simulink model "sampleModel1455"  (R2023a)
settings: Solver=VariableStepAuto  StartTime=0.0  StopTime=10.0  RelTol=1e-3
libraries: hdlsllib x5, simulink x3
settings Model: Creator=user1  LastModifiedBy=user1

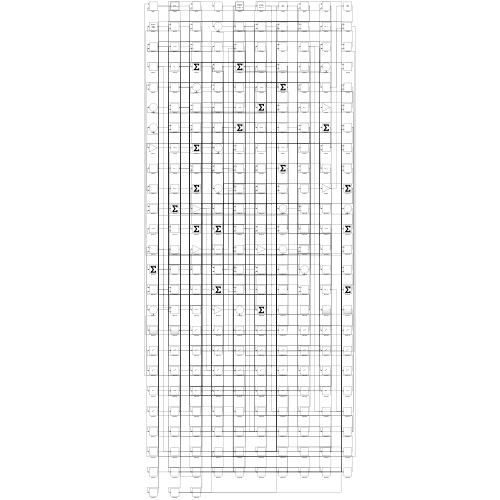
[thumbnail: Simulink's stored preview of the top-level diagram]
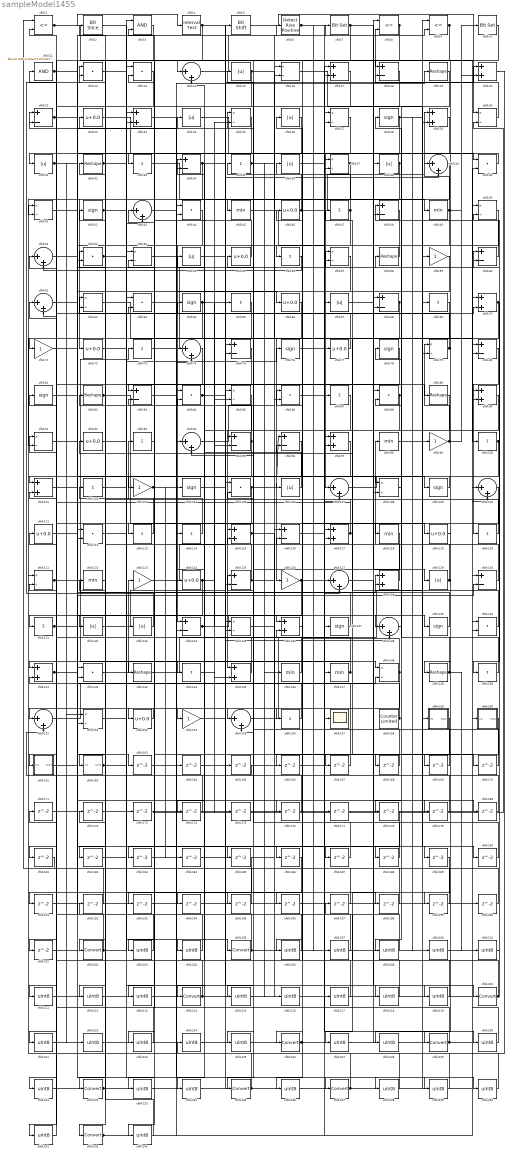
== system sampleModel1455 ==
  cfblk1 : RelationalOperator  Operator=<=  OutDataTypeStr=boolean  InputSameDT=off
  cfblk10 : simulink/Logic and Bit Operations/Bit Set  iBit=0
      settings: LibrarySourceBlock=|
      | hdlsllib/Logic and Bit
      | Operations/Bit Set
  cfblk{33,35,47,56,65,69,73,87,93,100,102,113..114,120,131,144,150,156} (18 alike) : Sum  Inputs=+
  cfblk{17,20,23,29,70,90,97,101,115,117,128,136,141,145} (14 alike) : Sum
  cfblk{59,71,99,103,123,126,154} (7 alike) : Gain
  cfblk{28,42,64,76,78,81,104,109,137,139} (10 alike) : Signum
  cfblk{12..13,40,44,52,63,84,86,88,105,112,140,142} (13 alike) : DotProduct  OutDataTypeStr=Inherit: Inherit via internal rule
  cfblk{15,24,26,31,36,38,54,67,106,129,132..133} (12 alike) : Abs  SaturateOnIntegerOverflow=off
  cfblk{14,39,43,51,61,74,94,107,110,127,138,151,155} (13 alike) : Sum  Inputs=|++
  cfblk{16,25,27,30,37,41,50,53,57,62,79,85,91,108,121,135,148,152} (18 alike) : Product  Inputs=*/  RndMeth=Zero  SaturateOnIntegerOverflow=on
  cfblk11 : simulink/Logic and Bit Operations/Bitwise Operator  logicop=AND  UseBitMask=on  BitMask=bin2dec('11011001')  BitMaskRealWorld=Stored Integer
      settings: LibrarySourceBlock=|
      | hdlsllib/Logic and Bit
      | Operations/Bitwise
      | Operator
  cfblk{22,46,55,66,72,77,92,111,119,124,153} (11 alike) : Bias  Bias=0.0  SaturateOnIntegerOverflow=off
  cfblk{18,21,34,48,60,68,75,80,83,95..96,116,125,130,134} (15 alike) : Sum  Inputs=+-
  cfblk{45,49,98,118,122,146..147} (7 alike) : MinMax
  cfblk{19,32,58,82,89,143,149} (7 alike) : Reshape
  cfblk157 : Scope
  cfblk158 : hdlsllib/Sources/Counter Limited  uplimit=7  tsamp=-1
  cfblk159 : Subsystem
      settings: LibrarySourceBlock=|
      | hdlsllib/Ports &
      | Subsystems/Subsystem
  cfblk160 : Subsystem
      settings: LibrarySourceBlock=|
      | hdlsllib/Ports &
      | Subsystems/Subsystem
  cfblk161 : Subsystem
      settings: LibrarySourceBlock=|
      | hdlsllib/Ports &
      | Subsystems/Subsystem
  cfblk162 : Subsystem
      settings: LibrarySourceBlock=|
      | hdlsllib/Ports &
      | Subsystems/Subsystem
  cfblk{163..201} (39 alike) : Delay  SampleTime=1
  cfblk2 : hdlsllib/Logic and Bit Operations/Bit Slice  lidx=7  ridx=0
  cfblk{202,205,214,220,226,229,232,235,237,242} (10 alike) : DataTypeConversion  SaturateOnIntegerOverflow=off  RndMeth=Floor
  cfblk{203..204,206..213,215..219,221..225,227..228,230..231,233..234,236,238..241,243} (32 alike) : DataTypeConversion  OutDataTypeStr=uint8  SaturateOnIntegerOverflow=off  RndMeth=Floor
  cfblk3 : Logic  AllPortsSameDT=off  OutDataTypeStr=boolean
  cfblk4 : hdlsllib/Logic and Bit Operations/Interval Test  IntervalClosedRight=on  uplimit=0.5  IntervalClosedLeft=on  lowlimit=-0.5  OutDataTypeStr=boolean
  cfblk5 : hdlsllib/Logic and Bit Operations/Bit Shift  mode=Shift Left Logical  N=0
  cfblk6 : hdlsllib/Logic and Bit Operations/Detect Rise Positive  vinit=0  OutDataTypeStr=boolean
  cfblk7 : simulink/Logic and Bit Operations/Bit Set  iBit=0
      settings: LibrarySourceBlock=|
      | hdlsllib/Logic and Bit
      | Operations/Bit Set
  cfblk8 : RelationalOperator  Operator=<=  OutDataTypeStr=boolean  InputSameDT=off
  cfblk9 : RelationalOperator  Operator=<=  OutDataTypeStr=boolean  InputSameDT=off
  wires:
  cfblk55/1 -> cfblk21/1
  cfblk14/1 -> cfblk7/1
  cfblk82/1 -> cfblk119/1, cfblk76/1
  cfblk66/1 -> cfblk126/1
  cfblk58/1 -> cfblk56/1
  cfblk40/1 -> cfblk33/1
  cfblk139/1 -> cfblk73/1
  cfblk63/1 -> cfblk205/1
  cfblk130/1 -> cfblk98/1
  cfblk73/1 -> cfblk35/1
  cfblk106/1 -> cfblk82/1
  cfblk89/1 -> cfblk145/1
  cfblk5/1 -> cfblk30/1
  cfblk133/1 -> cfblk12/1
  cfblk31/1 -> cfblk40/1, cfblk222/1
  cfblk70/1 -> cfblk150/1, cfblk112/2
  cfblk11/1 -> cfblk71/1, cfblk186/1
  cfblk102/1 -> cfblk237/1
  cfblk8/1 -> cfblk115/1, cfblk161/1(In1)
  cfblk22/1 -> cfblk107/1
  cfblk24/1 -> cfblk147/1
  cfblk47/1 -> cfblk142/2, cfblk15/1
  cfblk68/1 -> cfblk166/1, cfblk167/1
  cfblk100/1 -> cfblk134/1, cfblk206/1
  cfblk138/1 -> cfblk78/1
  cfblk57/1 -> cfblk114/1
  cfblk10/1 -> cfblk149/1
  cfblk44/1 -> cfblk94/1
  cfblk2/1 -> cfblk53/1
  cfblk17/1 -> cfblk45/1
  cfblk43/1 -> cfblk19/1
  cfblk15/1 -> cfblk31/1, cfblk18/1, cfblk49/1
  cfblk142/1 -> cfblk123/1
  cfblk109/1 -> cfblk101/1
  cfblk94/1 -> cfblk16/1
  cfblk149/1 -> cfblk128/1, cfblk210/1
  cfblk120/1 -> cfblk12/2
  cfblk99/1 -> cfblk79/1, cfblk20/2
  cfblk111/1 -> cfblk24/1
  cfblk117/1 -> cfblk93/1, cfblk91/1
  cfblk101/1 -> cfblk6/1
  cfblk59/1 -> cfblk235/1
  cfblk134/1 -> cfblk136/1, cfblk95/2
  cfblk37/1 -> cfblk72/1, cfblk52/2, cfblk212/1
  cfblk125/1 -> cfblk60/1, cfblk14/2
  cfblk123/1 -> cfblk5/1
  cfblk145/1 -> cfblk11/1
  cfblk155/1 -> cfblk38/1
  cfblk3/1 -> cfblk202/1
  cfblk121/1 -> cfblk143/1, cfblk152/1
  cfblk137/1 -> cfblk55/1
  cfblk98/1 -> cfblk69/1
  cfblk49/1 -> cfblk83/1, cfblk39/1, cfblk10/1
  cfblk46/1 -> cfblk29/1, cfblk25/1
  cfblk110/1 -> cfblk226/1
  cfblk136/1 -> cfblk26/1
  cfblk140/1 -> cfblk92/1
  cfblk6/1 -> cfblk37/2, cfblk207/1
  cfblk60/1 -> cfblk48/1
  cfblk113/1 -> cfblk52/1
  cfblk28/1 -> cfblk132/1, cfblk190/1, cfblk209/1
  cfblk29/1 -> cfblk48/2
  cfblk80/1 -> cfblk120/1
  cfblk105/1 -> cfblk96/1, cfblk221/1
  cfblk143/1 -> cfblk29/2
  cfblk78/1 -> cfblk113/1
  cfblk72/1 -> cfblk23/2
  cfblk84/1 -> cfblk18/2, cfblk175/1
  cfblk48/1 -> cfblk68/2
  cfblk64/1 -> cfblk85/2, cfblk91/2, cfblk39/2, cfblk193/1
  cfblk71/1 -> cfblk103/1
  cfblk132/1 -> cfblk65/1
  cfblk147/1 -> cfblk141/1, cfblk54/1
  cfblk1/1 -> cfblk100/1, cfblk4/1
  cfblk67/1 -> cfblk88/1
  cfblk62/1 -> cfblk99/1
  cfblk34/1 -> cfblk44/2, cfblk124/1, cfblk138/2
  cfblk124/1 -> cfblk25/2, cfblk201/1
  cfblk32/1 -> cfblk89/1, cfblk187/1, cfblk188/1
  cfblk45/1 -> cfblk107/2
  cfblk126/1 -> cfblk87/1, cfblk234/1
  cfblk42/1 -> cfblk2/1, cfblk108/1, cfblk179/1, cfblk180/1
  cfblk107/1 -> cfblk109/1
  cfblk135/1 -> cfblk9/2
  cfblk103/1 -> cfblk184/1, cfblk185/1
  cfblk33/1 -> cfblk157/1
  cfblk79/1 -> cfblk51/1, cfblk34/1
  cfblk30/1 -> cfblk8/2
  cfblk150/1 -> cfblk64/1
  cfblk93/1 -> cfblk43/1
  cfblk153/1 -> cfblk151/1
  cfblk13/1 -> cfblk162/1(In1)
  cfblk95/1 -> cfblk83/2, cfblk233/1
  cfblk81/1 -> cfblk58/1
  cfblk35/1 -> cfblk95/1, cfblk80/2, cfblk146/1
  cfblk97/1 -> cfblk214/1
  cfblk7/1 -> cfblk129/1, cfblk152/2
  cfblk56/1 -> cfblk51/2
  cfblk156/1 -> cfblk125/1
  cfblk144/1 -> cfblk145/2
  cfblk69/1 -> cfblk77/1
  cfblk9/1 -> cfblk156/1, cfblk125/2, cfblk213/1
  cfblk141/1 -> cfblk128/2, cfblk148/2, cfblk181/1
  cfblk128/1 -> cfblk42/1
  cfblk146/1 -> cfblk22/1
  cfblk131/1 -> cfblk130/2, cfblk176/1
  cfblk38/1 -> cfblk154/1, cfblk41/2
  cfblk19/1 -> cfblk118/1
  cfblk87/1 -> cfblk144/1
  cfblk118/1 -> cfblk155/1
  cfblk77/1 -> cfblk36/1
  cfblk148/1 -> cfblk46/1, cfblk182/1
  cfblk54/1 -> cfblk20/1
  cfblk96/1 -> cfblk153/1
  cfblk52/1 -> cfblk148/1, cfblk108/2, cfblk194/1
  cfblk21/1 -> cfblk139/1, cfblk66/1
  cfblk158/1 -> cfblk101/2, cfblk141/2
  cfblk115/1 -> cfblk168/1, cfblk216/1
  cfblk90/1 -> cfblk229/1
  cfblk92/1 -> cfblk57/1
  cfblk162/1(Out1) -> cfblk133/1, cfblk204/1
  cfblk114/1 -> cfblk62/1
  cfblk18/1 -> cfblk131/1
  cfblk151/1 -> cfblk137/1
  cfblk129/1 -> cfblk47/1, cfblk86/1, cfblk88/2
  cfblk161/1(Out1) -> cfblk70/2
  cfblk88/1 -> cfblk104/1, cfblk28/1
  cfblk16/1 -> cfblk159/1(In1)
  cfblk127/1 -> cfblk220/1
  cfblk91/1 -> cfblk138/1
  cfblk23/1 -> cfblk117/2
  cfblk75/1 -> cfblk232/1
  cfblk41/1 -> cfblk135/2
  cfblk122/1 -> cfblk242/1
  cfblk4/1 -> cfblk14/1, cfblk219/1
  cfblk51/1 -> cfblk163/1
  cfblk163/1 -> cfblk134/2
  cfblk164/1 -> cfblk57/2
  cfblk154/1 -> cfblk165/1
  cfblk165/1 -> cfblk151/2
  cfblk166/1 -> cfblk37/1
  cfblk167/1 -> cfblk1/2
  cfblk168/1 -> cfblk94/2
  cfblk119/1 -> cfblk169/1
  cfblk169/1 -> cfblk96/2
  cfblk76/1 -> cfblk170/1
  cfblk170/1 -> cfblk21/2
  cfblk171/1 -> cfblk140/1
  cfblk172/1 -> cfblk43/2
  cfblk173/1 -> cfblk30/2
  cfblk85/1 -> cfblk174/1
  cfblk174/1 -> cfblk53/2
  cfblk176/1 -> cfblk115/2
  cfblk36/1 -> cfblk177/1
  cfblk177/1 -> cfblk79/2
  cfblk108/1 -> cfblk178/1
  cfblk179/1 -> cfblk62/2
  cfblk180/1 -> cfblk34/2
  cfblk181/1 -> cfblk1/1
  cfblk182/1 -> cfblk13/1
  cfblk25/1 -> cfblk183/1
  cfblk183/1 -> cfblk44/1
  cfblk184/1 -> cfblk16/2
  cfblk187/1 -> cfblk155/2
  cfblk188/1 -> cfblk105/2
  cfblk104/1 -> cfblk189/1
  cfblk190/1 -> cfblk17/1
  cfblk65/1 -> cfblk191/1
  cfblk191/1 -> cfblk9/1
  cfblk192/1 -> cfblk142/1
  cfblk193/1 -> cfblk70/1
  cfblk194/1 -> cfblk117/1
  cfblk152/1 -> cfblk195/1
  cfblk195/1 -> cfblk121/2
  cfblk112/1 -> cfblk196/1
  cfblk196/1 -> cfblk8/1
  cfblk197/1 -> cfblk135/1
  cfblk83/1 -> cfblk198/1
  cfblk198/1 -> cfblk23/1
  cfblk160/1(Out1) -> cfblk199/1
  cfblk199/1 -> cfblk41/1
  cfblk200/1 -> cfblk136/2
  cfblk202/1 -> cfblk173/1, cfblk111/1
  cfblk178/1 -> cfblk203/1
  cfblk203/1 -> cfblk3/1
  cfblk204/1 -> cfblk3/2
  cfblk205/1 -> cfblk130/1, cfblk112/1
  cfblk206/1 -> cfblk63/1
  cfblk207/1 -> cfblk63/2
  cfblk50/1 -> cfblk208/1
  cfblk208/1 -> cfblk192/1
  cfblk209/1 -> cfblk50/1
  cfblk210/1 -> cfblk50/2
  cfblk74/1 -> cfblk211/1
  cfblk211/1 -> cfblk160/1(In1)
  cfblk212/1 -> cfblk74/1
  cfblk213/1 -> cfblk74/2
  cfblk214/1 -> cfblk171/1, cfblk86/2, cfblk106/1
  cfblk175/1 -> cfblk215/1
  cfblk215/1 -> cfblk97/1
  cfblk216/1 -> cfblk97/2
  cfblk116/1 -> cfblk217/1
  cfblk217/1 -> cfblk172/1
  cfblk12/1 -> cfblk218/1
  cfblk218/1 -> cfblk116/1
  cfblk219/1 -> cfblk116/2
  cfblk220/1 -> cfblk197/1, cfblk84/2, cfblk60/2
  cfblk221/1 -> cfblk127/1
  cfblk222/1 -> cfblk127/2
  cfblk27/1 -> cfblk223/1
  cfblk223/1 -> cfblk32/1
  cfblk20/1 -> cfblk224/1
  cfblk224/1 -> cfblk27/1
  cfblk186/1 -> cfblk225/1
  cfblk225/1 -> cfblk27/2
  cfblk226/1 -> cfblk67/1, cfblk68/1
  cfblk189/1 -> cfblk227/1
  cfblk227/1 -> cfblk110/1
  cfblk228/1 -> cfblk110/2
  cfblk229/1 -> cfblk228/1, cfblk81/1, cfblk13/2
  cfblk86/1 -> cfblk230/1
  cfblk230/1 -> cfblk90/1
  cfblk185/1 -> cfblk231/1
  cfblk231/1 -> cfblk90/2
  cfblk232/1 -> cfblk140/2, cfblk40/2
  cfblk233/1 -> cfblk75/1
  cfblk234/1 -> cfblk75/2
  cfblk235/1 -> cfblk80/1, cfblk121/1
  cfblk39/1 -> cfblk236/1
  cfblk236/1 -> cfblk59/1
  cfblk237/1 -> cfblk84/1, cfblk85/1
  cfblk53/1 -> cfblk238/1
  cfblk238/1 -> cfblk102/1
  cfblk61/1 -> cfblk239/1
  cfblk239/1 -> cfblk105/1
  cfblk201/1 -> cfblk240/1
  cfblk240/1 -> cfblk61/1
  cfblk26/1 -> cfblk241/1
  cfblk241/1 -> cfblk61/2
  cfblk242/1 -> cfblk200/1, cfblk164/1, cfblk17/2
  cfblk159/1(Out1) -> cfblk243/1
  cfblk243/1 -> cfblk122/1

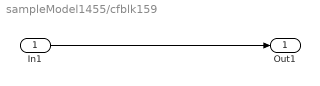
== system sampleModel1455/cfblk159 ==
  In1 : Inport
  Out1 : Outport
  wires:
  In1/1 -> Out1/1

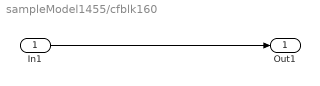
== system sampleModel1455/cfblk160 ==
  In1 : Inport
  Out1 : Outport
  wires:
  In1/1 -> Out1/1

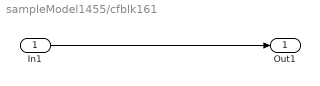
== system sampleModel1455/cfblk161 ==
  In1 : Inport
  Out1 : Outport
  wires:
  In1/1 -> Out1/1

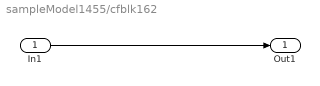
== system sampleModel1455/cfblk162 ==
  In1 : Inport
  Out1 : Outport
  wires:
  In1/1 -> Out1/1
